simulink model "processor_with_peripherals"  (R2025a)
settings: Solver=FixedStepDiscrete  StartTime=0.0  StopTime=inf  RelTol=1e-3
libraries: simulink x6
(part 3 of 5)

== system processor_with_peripherals/SysTick_Timer ==
  In1 : Inport
  In2 : Inport  Port=2
  RAM_WData : Inport  Port=3
  Compare To Constant : simulink/Logic and Bit Operations/Compare To Constant  relop===  const=-16  OutDataTypeStr=boolean
  Counter Free-Running : simulink/Sources/Counter Free-Running  NumBits=16  tsamp=1
  Logical Operator : Logic  AllPortsSameDT=off  OutDataTypeStr=boolean
  Relational Operator : RelationalOperator  Operator===  OutDataTypeStr=boolean  RndMeth=Simplest  InputSameDT=off
  Scope : Scope
      settings: ActiveDisplayYMinimum=-1  ActiveDisplayYMaximum=1  DataLoggingVariableName=ScopeData7
  Switch : Switch  Criteria=u2 > Threshold  SaturateOnIntegerOverflow=off  InputSameDT=off
  Unit Delay : UnitDelay  InitialCondition=10000  HasFrameUpgradeWarning=on
  Out1 : Outport
  wires:
  In1/1 -> Compare To Constant/1  "Address"
  In2/1 -> Logical Operator/2  "MemWrite"
  RAM_WData/1 -> Switch/1  "WriteData"
  Relational Operator/1 -> Scope/1, Out1/1  "IRQ_Out"
  Compare To Constant/1 -> Logical Operator/1
  Unit Delay/1 -> Relational Operator/1, Switch/3
  Switch/1 -> Unit Delay/1
  Counter Free-Running/1 -> Relational Operator/2
  Logical Operator/1 -> Switch/2

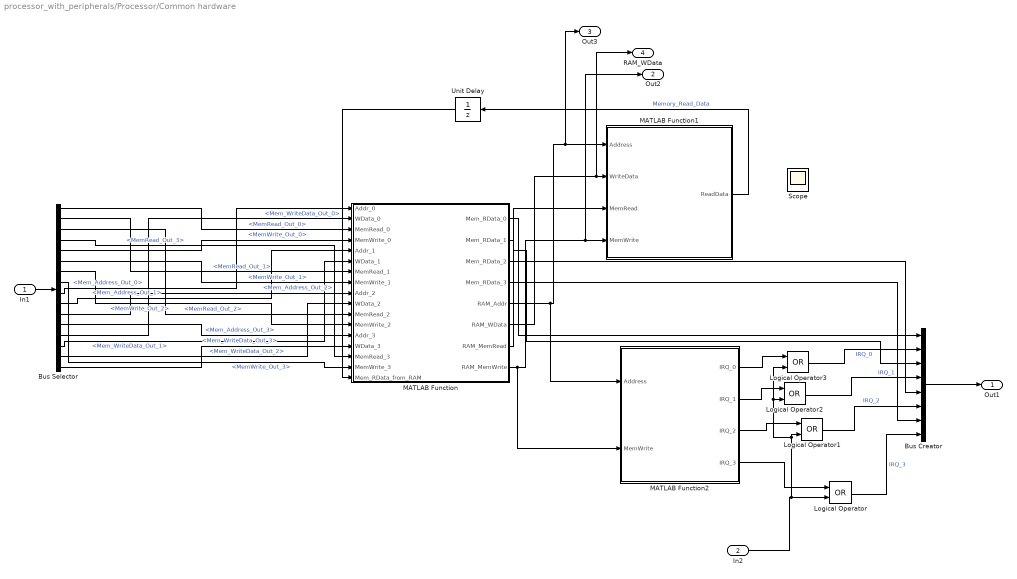
== system processor_with_peripherals/Processor/Common hardware ==
  In1 : Inport
  In2 : Inport  Port=2
  Bus Creator : BusCreator  Inputs=8  OutDataTypeStr=Bus: CH0_Bus
  Bus Selector : BusSelector  OutputSignals=MemRead_Out_0,MemRead_Out_1,MemRead_Out_2,MemRead_Out_3,MemWrite_Out_0,MemWrite_Out_1,MemWrite_Out_2,MemWrite_Out_3,Mem_Address_Out_0,Mem_Address_Out_1,Mem_Address_Out_2,Mem_Address_Out_3,Mem_WriteData_Out_0,Mem_WriteData_Out_1,Mem_WriteData_Out_2,Mem_WriteData_Out_3
  Logical Operator{,1..3} (4 alike) : Logic  Operator=OR  AllPortsSameDT=off  OutDataTypeStr=boolean
  MATLAB Function : MATLAB Function  TreatAsAtomicUnit=on
  MATLAB Function1 : MATLAB Function  TreatAsAtomicUnit=on
  MATLAB Function2 : MATLAB Function  TreatAsAtomicUnit=on
  Scope : Scope
      settings: ActiveDisplayYMinimum=-9.9596643418991722  ActiveDisplayYMaximum=10.040335658100835  DataLoggingVariableName=ScopeData3
  Unit Delay : UnitDelay  HasFrameUpgradeWarning=on
  Out1 : Outport
  Out2 : Outport  Port=2
  Out3 : Outport  Port=3
  RAM_WData : Outport  Port=4
  wires:
  MATLAB Function/5(RAM_Addr) -> MATLAB Function2/1(Address), Out3/1, MATLAB Function1/1(Address)
  MATLAB Function/6(RAM_WData) -> RAM_WData/1, MATLAB Function1/2(WriteData)
  MATLAB Function/7(RAM_MemRead) -> MATLAB Function1/3(MemRead)
  MATLAB Function/8(RAM_MemWrite) -> Out2/1, MATLAB Function1/4(MemWrite), MATLAB Function2/2(MemWrite)
  MATLAB Function1/1(ReadData) -> Unit Delay/1  "Memory_Read_Data"
  MATLAB Function/1(Mem_RData_0) -> Bus Creator/1
  MATLAB Function2/1(IRQ_0) -> Logical Operator3/1
  MATLAB Function/2(Mem_RData_1) -> Bus Creator/3
  MATLAB Function/3(Mem_RData_2) -> Bus Creator/5
  MATLAB Function2/3(IRQ_2) -> Logical Operator1/1
  MATLAB Function/4(Mem_RData_3) -> Bus Creator/7
  MATLAB Function2/4(IRQ_3) -> Logical Operator/1
  In1/1 -> Bus Selector/1
  Bus Creator/1 -> Out1/1
  Bus Selector/1 -> MATLAB Function/3(MemRead_0)  "<MemRead_Out_0>"
  Bus Selector/2 -> MATLAB Function/7(MemRead_1)  "<MemRead_Out_1>"
  Bus Selector/3 -> MATLAB Function/11(MemRead_2)  "<MemRead_Out_2>"
  Bus Selector/4 -> MATLAB Function/15(MemRead_3)  "<MemRead_Out_3>"
  Bus Selector/5 -> MATLAB Function/4(MemWrite_0)  "<MemWrite_Out_0>"
  Bus Selector/6 -> MATLAB Function/8(MemWrite_1)  "<MemWrite_Out_1>"
  Bus Selector/7 -> MATLAB Function/12(MemWrite_2)  "<MemWrite_Out_2>"
  Bus Selector/8 -> MATLAB Function/16(MemWrite_3)  "<MemWrite_Out_3>"
  Bus Selector/9 -> MATLAB Function/1(Addr_0)  "<Mem_Address_Out_0>"
  Bus Selector/10 -> MATLAB Function/5(Addr_1)  "<Mem_Address_Out_1>"
  Bus Selector/11 -> MATLAB Function/9(Addr_2)  "<Mem_Address_Out_2>"
  Bus Selector/12 -> MATLAB Function/13(Addr_3)  "<Mem_Address_Out_3>"
  Bus Selector/13 -> MATLAB Function/2(WData_0)  "<Mem_WriteData_Out_0>"
  Bus Selector/14 -> MATLAB Function/6(WData_1)  "<Mem_WriteData_Out_1>"
  Bus Selector/15 -> MATLAB Function/10(WData_2)  "<Mem_WriteData_Out_2>"
  Bus Selector/16 -> MATLAB Function/14(WData_3)  "<Mem_WriteData_Out_3>"
  Unit Delay/1 -> MATLAB Function/17(Mem_RData_from_RAM)
  Logical Operator/1 -> Bus Creator/8  "IRQ_3"
  Logical Operator1/1 -> Bus Creator/6  "IRQ_2"
  MATLAB Function2/2(IRQ_1) -> Logical Operator2/1
  Logical Operator2/1 -> Bus Creator/4  "IRQ_1"
  Logical Operator3/1 -> Bus Creator/2  "IRQ_0"
  In2/1 -> Logical Operator3/2, Logical Operator2/2, Logical Operator1/2, Logical Operator/2

== system processor_with_peripherals/Processor/Core_0 ==
  In1 : Inport
  In2 : Inport  Port=2
  Bus Creator : BusCreator  Inputs=10  OutDataTypeStr=Bus: C01_Bus
  Bus Selector : BusSelector  OutputSignals=Mem_RData_0,IRQ_0,Mem_RData_1,IRQ_1,Mem_RData_2,IRQ_2,Mem_RData_3,IRQ_3
  EX/MEM Pipeline Register : UnitDelay  HasFrameUpgradeWarning=on
  Execute (EX) Stage : Subsystem
  ID/EX Pipeline Register : UnitDelay  HasFrameUpgradeWarning=on
  IF/ID Pipeline Register : UnitDelay  HasFrameUpgradeWarning=on
  Instruction Decode(ID) Stage : Subsystem
  Instruction Fetch (IF) Stage : Subsystem
  MEM/WB Pipeline Register : UnitDelay  HasFrameUpgradeWarning=on
  Memory Access : Subsystem
  Write Back : Subsystem
  Out1 : Outport
  Out2 : Outport  Port=2
  wires:
  IF/ID Pipeline Register/1 -> Instruction Decode(ID) Stage/1(In1)
  Instruction Decode(ID) Stage/1(Out1) -> ID/EX Pipeline Register/1
  MEM/WB Pipeline Register/1 -> Write Back/1(In1)
  Memory Access/1(Out1) -> MEM/WB Pipeline Register/1
  Instruction Fetch (IF) Stage/1(Out1) -> IF/ID Pipeline Register/1
  EX/MEM Pipeline Register/1 -> Memory Access/1(In1)
  Execute (EX) Stage/1(Out1) -> EX/MEM Pipeline Register/1
  ID/EX Pipeline Register/1 -> Execute (EX) Stage/1(In1)
  Write Back/1(Out1) -> Instruction Decode(ID) Stage/2(In2)
  Instruction Fetch (IF) Stage/2(Out2) -> Out1/1  "Instruction_Address_Out"
  Memory Access/2(Out2) -> Bus Creator/3  "Mem_Address_Out_0"
  Memory Access/3(Out3) -> Bus Creator/2  "Mem_WriteData_Out_0"
  Memory Access/4(Out4) -> Bus Creator/1  "MemRead_Out_0"
  Memory Access/5(Out5) -> Bus Creator/4  "MemWrite_Out_0"
  Bus Selector/1 -> Write Back/2(In2)  "<Mem_RData_0>"
  In1/1 -> Bus Selector/1
  Bus Selector/2 -> Instruction Fetch (IF) Stage/2(In2)  "<IRQ_0>"
  Bus Creator/1 -> Out2/1
  Bus Selector/3 -> Bus Creator/5  "<Mem_RData_1>"
  Bus Selector/4 -> Bus Creator/6  "<IRQ_1>"
  Bus Selector/5 -> Bus Creator/7  "<Mem_RData_2>"
  Bus Selector/6 -> Bus Creator/8  "<IRQ_2>"
  Bus Selector/7 -> Bus Creator/9  "<Mem_RData_3>"
  Bus Selector/8 -> Bus Creator/10  "<IRQ_3>"
  In2/1 -> Instruction Fetch (IF) Stage/1(In1)

== system processor_with_peripherals/Processor/Core_1 ==
  In2 : Inport
  In1 : Inport  Port=2
  Bus Creator : BusCreator  Inputs=12  OutDataTypeStr=Bus: C12_Bus
  Bus Selector : BusSelector  OutputSignals=IRQ_1,Mem_RData_1,MemWrite_Out_0,Mem_Address_Out_0,Mem_WriteData_Out_0,MemRead_Out_0,Mem_RData_2,IRQ_2,Mem_RData_3,IRQ_3
  EX/MEM Pipeline Register : UnitDelay  HasFrameUpgradeWarning=on
  Execute (EX) Stage : Subsystem
  ID/EX Pipeline Register : UnitDelay  HasFrameUpgradeWarning=on
  IF/ID Pipeline Register : UnitDelay  HasFrameUpgradeWarning=on
  Instruction Decode(ID) Stage : Subsystem
  Instruction Fetch (IF) Stage : Subsystem
  MEM/WB Pipeline Register : UnitDelay  HasFrameUpgradeWarning=on
  Memory Access : Subsystem
  Write Back : Subsystem
  Out1 : Outport
  Out2 : Outport  Port=2
  wires:
  IF/ID Pipeline Register/1 -> Instruction Decode(ID) Stage/1(In1)
  Instruction Decode(ID) Stage/1(Out1) -> ID/EX Pipeline Register/1
  MEM/WB Pipeline Register/1 -> Write Back/1(In1)
  Memory Access/1(Out1) -> MEM/WB Pipeline Register/1
  Instruction Fetch (IF) Stage/1(Out1) -> IF/ID Pipeline Register/1
  EX/MEM Pipeline Register/1 -> Memory Access/1(In1)
  Execute (EX) Stage/1(Out1) -> EX/MEM Pipeline Register/1
  ID/EX Pipeline Register/1 -> Execute (EX) Stage/1(In1)
  Write Back/1(Out1) -> Instruction Decode(ID) Stage/2(In2)
  Instruction Fetch (IF) Stage/2(Out2) -> Out1/1  "Instruction_Address_Out"
  Memory Access/2(Out2) -> Bus Creator/3  "Mem_Address_Out_1"
  Memory Access/3(Out3) -> Bus Creator/2  "Mem_WriteData_Out_1"
  Memory Access/4(Out4) -> Bus Creator/1  "MemRead_Out_1"
  Memory Access/5(Out5) -> Bus Creator/4  "MemWrite_Out_1"
  In2/1 -> Bus Selector/1
  Bus Creator/1 -> Out2/1
  In1/1 -> Instruction Fetch (IF) Stage/1(In1)
  Bus Selector/1 -> Instruction Fetch (IF) Stage/2(In2)  "<IRQ_1>"
  Bus Selector/2 -> Write Back/2(In2)  "<Mem_RData_1>"
  Bus Selector/3 -> Bus Creator/5  "<MemWrite_Out_0>"
  Bus Selector/4 -> Bus Creator/6  "<Mem_Address_Out_0>"
  Bus Selector/5 -> Bus Creator/7  "<Mem_WriteData_Out_0>"
  Bus Selector/6 -> Bus Creator/8  "<MemRead_Out_0>"
  Bus Selector/7 -> Bus Creator/9  "<Mem_RData_2>"
  Bus Selector/8 -> Bus Creator/10  "<IRQ_2>"
  Bus Selector/9 -> Bus Creator/11  "<Mem_RData_3>"
  Bus Selector/10 -> Bus Creator/12  "<IRQ_3>"

== system processor_with_peripherals/Processor/Core_2 ==
  In1 : Inport
  In2 : Inport  Port=2
  Bus Creator : BusCreator  Inputs=14  OutDataTypeStr=Bus: C23_Bus
  Bus Selector : BusSelector  OutputSignals=Mem_RData_2,IRQ_2,MemRead_Out_1,Mem_WriteData_Out_1,Mem_Address_Out_1,MemWrite_Out_1,MemWrite_Out_0,Mem_Address_Out_0,Mem_WriteData_Out_0,MemRead_Out_0,Mem_RData_3,IRQ_3
  EX/MEM Pipeline Register : UnitDelay  HasFrameUpgradeWarning=on
  Execute (EX) Stage : Subsystem
  ID/EX Pipeline Register : UnitDelay  HasFrameUpgradeWarning=on
  IF/ID Pipeline Register : UnitDelay  HasFrameUpgradeWarning=on
  Instruction Decode(ID) Stage : Subsystem
  Instruction Fetch (IF) Stage : Subsystem
  MEM/WB Pipeline Register : UnitDelay  HasFrameUpgradeWarning=on
  Memory Access : Subsystem
  Write Back : Subsystem
  Out1 : Outport
  Out2 : Outport  Port=2
  wires:
  IF/ID Pipeline Register/1 -> Instruction Decode(ID) Stage/1(In1)
  Instruction Decode(ID) Stage/1(Out1) -> ID/EX Pipeline Register/1
  MEM/WB Pipeline Register/1 -> Write Back/1(In1)
  Memory Access/1(Out1) -> MEM/WB Pipeline Register/1
  Instruction Fetch (IF) Stage/1(Out1) -> IF/ID Pipeline Register/1
  EX/MEM Pipeline Register/1 -> Memory Access/1(In1)
  Execute (EX) Stage/1(Out1) -> EX/MEM Pipeline Register/1
  ID/EX Pipeline Register/1 -> Execute (EX) Stage/1(In1)
  Write Back/1(Out1) -> Instruction Decode(ID) Stage/2(In2)
  In1/1 -> Instruction Fetch (IF) Stage/1(In1)  "Instruction_In"
  Instruction Fetch (IF) Stage/2(Out2) -> Out1/1  "Instruction_Address_Out"
  Memory Access/2(Out2) -> Bus Creator/3  "Mem_Address_Out_2"
  Memory Access/3(Out3) -> Bus Creator/2  "Mem_WriteData_Out_2"
  Memory Access/4(Out4) -> Bus Creator/1  "MemRead_Out_2"
  Memory Access/5(Out5) -> Bus Creator/4  "MemWrite_Out_2"
  Bus Selector/1 -> Write Back/2(In2)  "<Mem_RData_2>"
  Bus Selector/2 -> Instruction Fetch (IF) Stage/2(In2)  "<IRQ_2>"
  In2/1 -> Bus Selector/1
  Bus Creator/1 -> Out2/1
  Bus Selector/3 -> Bus Creator/5  "<MemRead_Out_1>"
  Bus Selector/4 -> Bus Creator/6  "<Mem_WriteData_Out_1>"
  Bus Selector/5 -> Bus Creator/7  "<Mem_Address_Out_1>"
  Bus Selector/6 -> Bus Creator/8  "<MemWrite_Out_1>"
  Bus Selector/7 -> Bus Creator/9  "<MemWrite_Out_0>"
  Bus Selector/8 -> Bus Creator/10  "<Mem_Address_Out_0>"
  Bus Selector/9 -> Bus Creator/11  "<Mem_WriteData_Out_0>"
  Bus Selector/10 -> Bus Creator/12  "<MemRead_Out_0>"
  Bus Selector/11 -> Bus Creator/13  "<Mem_RData_3>"
  Bus Selector/12 -> Bus Creator/14  "<IRQ_3>"

== system processor_with_peripherals/Processor/Core_3 ==
  In1 : Inport
  In2 : Inport  Port=2
  Bus Creator : BusCreator  Inputs=16  OutDataTypeStr=Bus: C3CH_Bus
  Bus Selector : BusSelector  OutputSignals=IRQ_3,Mem_RData_3,MemRead_Out_1,MemWrite_Out_2,Mem_Address_Out_2,Mem_WriteData_Out_2,MemRead_Out_2,Mem_WriteData_Out_1,Mem_Address_Out_1,MemWrite_Out_1,MemWrite_Out_0,Mem_Address_Out_0,Mem_WriteData_Out_0,MemRead_Out_0
  EX/MEM Pipeline Register : UnitDelay  HasFrameUpgradeWarning=on
  Execute (EX) Stage : Subsystem
  ID/EX Pipeline Register : UnitDelay  HasFrameUpgradeWarning=on
  IF/ID Pipeline Register : UnitDelay  HasFrameUpgradeWarning=on
  Instruction Decode(ID) Stage : Subsystem
  Instruction Fetch (IF) Stage : Subsystem
  MEM/WB Pipeline Register : UnitDelay  HasFrameUpgradeWarning=on
  Memory Access : Subsystem
  Write Back : Subsystem
  Out1 : Outport
  Out2 : Outport  Port=2
  wires:
  IF/ID Pipeline Register/1 -> Instruction Decode(ID) Stage/1(In1)
  Instruction Decode(ID) Stage/1(Out1) -> ID/EX Pipeline Register/1
  MEM/WB Pipeline Register/1 -> Write Back/1(In1)
  Memory Access/1(Out1) -> MEM/WB Pipeline Register/1
  Instruction Fetch (IF) Stage/1(Out1) -> IF/ID Pipeline Register/1
  EX/MEM Pipeline Register/1 -> Memory Access/1(In1)
  Execute (EX) Stage/1(Out1) -> EX/MEM Pipeline Register/1
  ID/EX Pipeline Register/1 -> Execute (EX) Stage/1(In1)
  Write Back/1(Out1) -> Instruction Decode(ID) Stage/2(In2)
  In1/1 -> Instruction Fetch (IF) Stage/1(In1)  "Instruction_In"
  Instruction Fetch (IF) Stage/2(Out2) -> Out1/1  "Instruction_Address_Out"
  Memory Access/2(Out2) -> Bus Creator/3  "Mem_Address_Out_3"
  Memory Access/3(Out3) -> Bus Creator/2  "Mem_WriteData_Out_3"
  Memory Access/4(Out4) -> Bus Creator/1  "MemRead_Out_3"
  Memory Access/5(Out5) -> Bus Creator/4  "MemWrite_Out_3"
  Bus Selector/2 -> Write Back/2(In2)  "<Mem_RData_3>"
  In2/1 -> Bus Selector/1
  Bus Creator/1 -> Out2/1
  Bus Selector/1 -> Instruction Fetch (IF) Stage/2(In2)  "<IRQ_3>"
  Bus Selector/3 -> Bus Creator/5  "<MemRead_Out_1>"
  Bus Selector/4 -> Bus Creator/6  "<MemWrite_Out_2>"
  Bus Selector/5 -> Bus Creator/7  "<Mem_Address_Out_2>"
  Bus Selector/6 -> Bus Creator/8  "<Mem_WriteData_Out_2>"
  Bus Selector/7 -> Bus Creator/9  "<MemRead_Out_2>"
  Bus Selector/8 -> Bus Creator/10  "<Mem_WriteData_Out_1>"
  Bus Selector/9 -> Bus Creator/11  "<Mem_Address_Out_1>"
  Bus Selector/10 -> Bus Creator/12  "<MemWrite_Out_1>"
  Bus Selector/11 -> Bus Creator/13  "<MemWrite_Out_0>"
  Bus Selector/12 -> Bus Creator/14  "<Mem_Address_Out_0>"
  Bus Selector/13 -> Bus Creator/15  "<Mem_WriteData_Out_0>"
  Bus Selector/14 -> Bus Creator/16  "<MemRead_Out_0>"

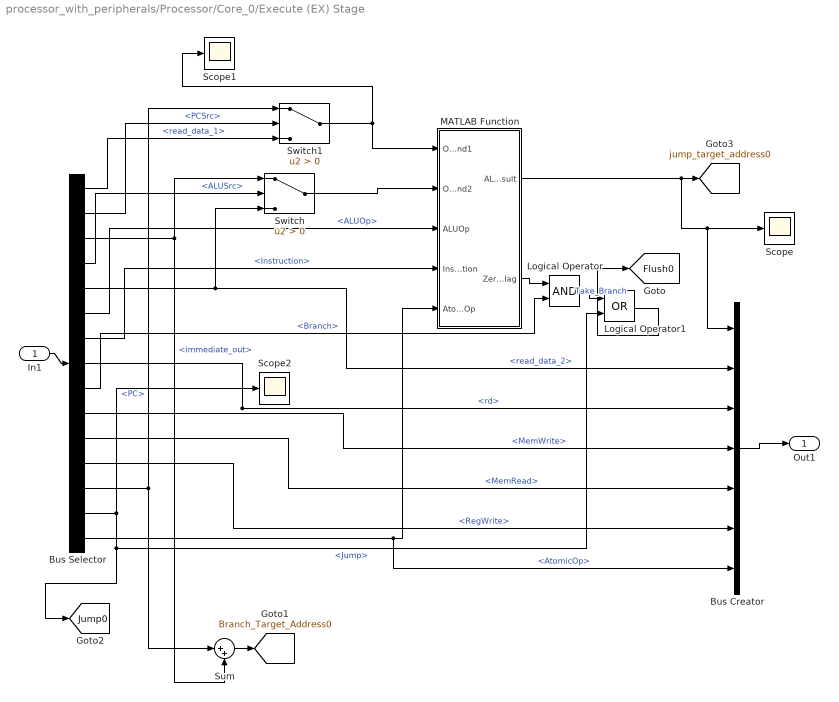
== system processor_with_peripherals/Processor/Core_0/Execute (EX) Stage ==
  In1 : Inport
  Bus Creator : BusCreator  Inputs=7  OutDataTypeStr=Bus: EXMEM_Bus  NonVirtualBus=on
  Bus Selector : BusSelector  OutputSignals=read_data_1,PCSrc,immediate_out,ALUSrc,read_data_2,ALUOp,Instruction,rd,Branch,MemWrite,MemRead,RegWrite,PC,Jump,AtomicOp
  Logical Operator : Logic  AllPortsSameDT=off  OutDataTypeStr=boolean
  Logical Operator1 : Logic  Operator=OR  AllPortsSameDT=off  OutDataTypeStr=boolean
  MATLAB Function : MATLAB Function  TreatAsAtomicUnit=on
  Scope : Scope
      settings: ActiveDisplayYMinimum=31.795159975888414  ActiveDisplayYMaximum=57.507794048249679
  Scope1 : Scope
      settings: ActiveDisplayYMinimum=91.787947621079041  ActiveDisplayYMaximum=102.5794088339111
  Scope2 : Scope
      settings: ActiveDisplayYMinimum=-11.618054609297872  ActiveDisplayYMaximum=8.6667189404735723  DataLoggingVariableName=ScopeData2
  Sum : Sum  Inputs=|++
  Switch : Switch  Criteria=u2 > Threshold  OutDataTypeStr=int32  SaturateOnIntegerOverflow=off  InputSameDT=off
  Switch1 : Switch  Criteria=u2 > Threshold  OutDataTypeStr=int32  SaturateOnIntegerOverflow=off  InputSameDT=off
  Out1 : Outport
  tag scope: Branch_Target_Address0=global, Flush0=global, Jump0=global, jump_target_address0=global
  wires:
  Bus Creator/1 -> Out1/1
  In1/1 -> Bus Selector/1
  Bus Selector/3 -> Sum/2, Switch/1  "<immediate_out>"
  Bus Selector/8 -> Bus Creator/3  "<rd>"
  Bus Selector/5 -> Bus Creator/2, Switch/3  "<read_data_2>"
  Bus Selector/1 -> Switch1/3  "<read_data_1>"
  Bus Selector/6 -> MATLAB Function/3(ALUOp)  "<ALUOp>"
  Bus Selector/14 -> [Jump0], Logical Operator1/2, Scope2/1  "<Jump>"
  Bus Selector/9 -> Logical Operator/2  "<Branch>"
  Bus Selector/10 -> Bus Creator/4  "<MemWrite>"
  Bus Selector/11 -> Bus Creator/5  "<MemRead>"
  Bus Selector/4 -> Switch/2  "<ALUSrc>"
  Bus Selector/12 -> Bus Creator/6  "<RegWrite>"
  Bus Selector/7 -> MATLAB Function/4(Instruction)  "<Instruction>"
  Switch/1 -> MATLAB Function/2(Operand2)
  MATLAB Function/1(ALU_Result) -> Scope/1, Bus Creator/1, [jump_target_address0]
  MATLAB Function/2(Zero_Flag) -> Logical Operator/1
  Logical Operator/1 -> Logical Operator1/1  "Take_Branch"
  Bus Selector/13 -> Sum/1, Switch1/1  "<PC>"
  Sum/1 -> [Branch_Target_Address0]
  Bus Selector/2 -> Switch1/2  "<PCSrc>"
  Switch1/1 -> Scope1/1, MATLAB Function/1(Operand1)
  Logical Operator1/1 -> [Flush0]
  Bus Selector/15 -> Bus Creator/7, MATLAB Function/5(AtomicOp)  "<AtomicOp>"

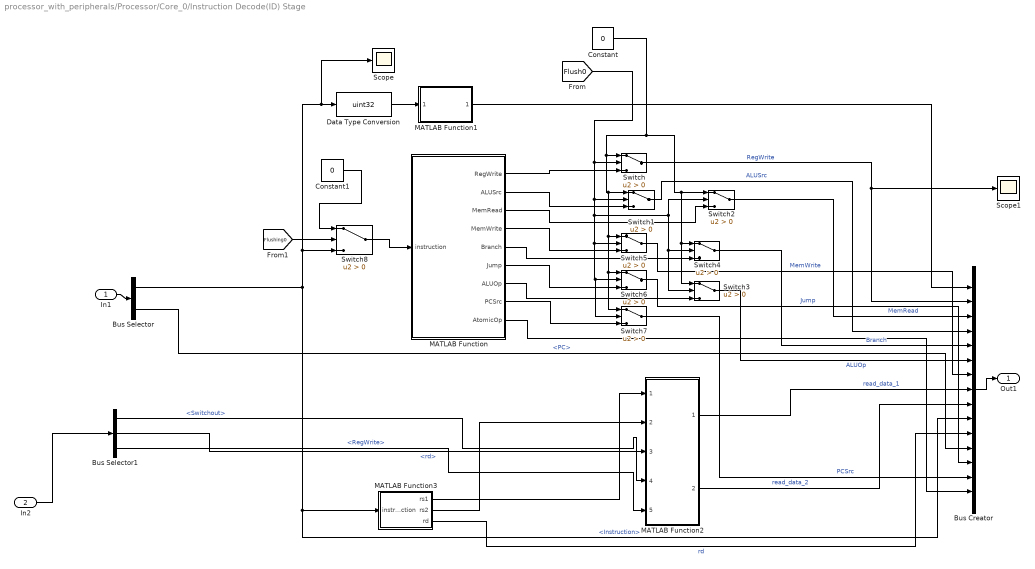
== system processor_with_peripherals/Processor/Core_0/Instruction Decode(ID) Stage ==
  In1 : Inport
  In2 : Inport  Port=2
  Bus Creator : BusCreator  Inputs=15  OutDataTypeStr=Bus: IDEX_Bus  NonVirtualBus=on
  Bus Selector : BusSelector  OutputSignals=Instruction,PC
  Bus Selector1 : BusSelector  OutputSignals=Switchout,rd,RegWrite
  Constant : Constant  Value=0  OutDataTypeStr=uint8
  Constant1 : Constant  Value=0
  Data Type Conversion : DataTypeConversion  OutDataTypeStr=uint32  SaturateOnIntegerOverflow=off  RndMeth=Floor
  MATLAB Function : MATLAB Function  TreatAsAtomicUnit=on
  MATLAB Function1 : MATLAB Function  TreatAsAtomicUnit=on
  MATLAB Function2 : MATLAB Function  TreatAsAtomicUnit=on
  MATLAB Function3 : MATLAB Function  TreatAsAtomicUnit=on
  Scope : Scope
      settings: ActiveDisplayYMinimum=-8.6059552101299882E+7  ActiveDisplayYMaximum=2.8669047582629967E+8  DataLoggingVariableName=ScopeData4
  Scope1 : Scope
      settings: ActiveDisplayYMinimum=-20.131283374012085  ActiveDisplayYMaximum=16.717122271781463  DataLoggingVariableName=ScopeData5
  Switch{,1..2,5..6} (5 alike) : Switch  Criteria=u2 > Threshold  OutDataTypeStr=boolean  SaturateOnIntegerOverflow=off  InputSameDT=off
  Switch3 : Switch  Criteria=u2 > Threshold  OutDataTypeStr=uint32  SaturateOnIntegerOverflow=off  InputSameDT=off
  Switch4 : Switch  Criteria=u2 > Threshold  OutDataTypeStr=uint32  SaturateOnIntegerOverflow=off  InputSameDT=off
  Switch7 : Switch  Criteria=u2 > Threshold  OutDataTypeStr=uint32  SaturateOnIntegerOverflow=off  InputSameDT=off
  Switch8 : Switch  Criteria=u2 > Threshold  SaturateOnIntegerOverflow=off  InputSameDT=off
  Out1 : Outport
  wires:
  Bus Creator/1 -> Out1/1
  In1/1 -> Bus Selector/1
  Bus Selector/1 -> Data Type Conversion/1, Scope/1, Switch8/3, MATLAB Function3/1(instruction), Bus Creator/10  "<Instruction>"
  MATLAB Function2/1(ReadData1) -> Bus Creator/8  "read_data_1"
  MATLAB Function2/2(ReadData2) -> Bus Creator/9  "read_data_2"
  MATLAB Function1/1(immediate_out) -> Bus Creator/1
  MATLAB Function3/3(rd) -> Bus Creator/11  "rd"
  MATLAB Function/7(ALUOp) -> Switch3/3
  MATLAB Function/6(Jump) -> Switch6/3
  MATLAB Function/5(Branch) -> Switch4/3
  MATLAB Function/4(MemWrite) -> Switch5/3
  MATLAB Function/3(MemRead) -> Switch2/3
  MATLAB Function/2(ALUSrc) -> Switch1/3
  Bus Selector1/2 -> MATLAB Function2/3(WriteAddr)  "<rd>"
  Bus Selector1/3 -> MATLAB Function2/5(WriteEnable)  "<RegWrite>"
  Bus Selector1/1 -> MATLAB Function2/4(WriteData)  "<Switchout>"
  MATLAB Function3/2(rs2) -> MATLAB Function2/2(ReadAddr2)
  Bus Selector/2 -> Bus Creator/12  "<PC>"
  MATLAB Function/8(PCSrc) -> Switch7/3
  MATLAB Function/1(RegWrite) -> Switch/3
  [Flush0] -> Switch1/2, Switch3/2, Switch4/2, Switch2/2, Switch7/2, Switch6/2, Switch5/2, Switch/2
  Constant/1 -> Switch3/1, Switch4/1, Switch2/1, Switch7/1, Switch6/1, Switch5/1, Switch1/1, Switch/1
  Switch/1 -> Scope1/1, Bus Creator/2  "RegWrite"
  Switch2/1 -> Bus Creator/3  "MemRead"
  Switch1/1 -> Bus Creator/4  "ALUSrc"
  Switch4/1 -> Bus Creator/5  "Branch"
  Switch3/1 -> Bus Creator/6  "ALUOp"
  Switch5/1 -> Bus Creator/7  "MemWrite"
  Switch6/1 -> Bus Creator/13  "Jump"
  Switch7/1 -> Bus Creator/14  "PCSrc"
  MATLAB Function3/1(rs1) -> MATLAB Function2/1(ReadAddr1)
  In2/1 -> Bus Selector1/1
  Switch8/1 -> MATLAB Function/1(instruction)
  Constant1/1 -> Switch8/1
  [Flushing0] -> Switch8/2
  Data Type Conversion/1 -> MATLAB Function1/1(instruction)
  MATLAB Function/9(AtomicOp) -> Bus Creator/15

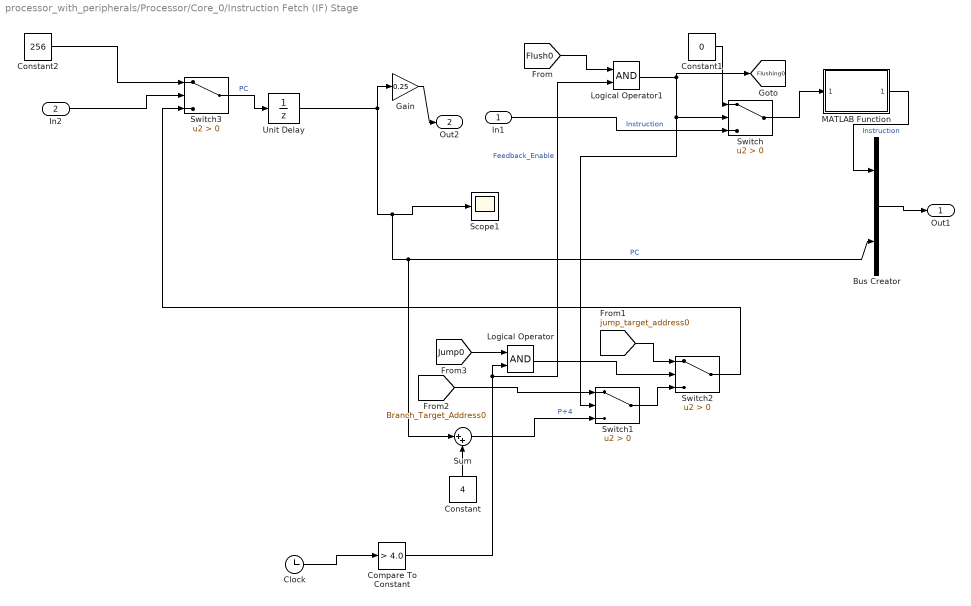
== system processor_with_peripherals/Processor/Core_0/Instruction Fetch (IF) Stage ==
  In1 : Inport
  In2 : Inport  Port=2
  Bus Creator : BusCreator  Inputs=2  OutDataTypeStr=Bus: IFID_Bus  NonVirtualBus=on
  Clock : Clock
  Compare To Constant : simulink/Logic and Bit Operations/Compare To Constant  relop=>  const=4.0  OutDataTypeStr=boolean
  Constant : Constant  Value=4
  Constant1 : Constant  Value=0
  Constant2 : Constant  Value=256  OutDataTypeStr=uint32
  Gain : Gain  Gain=0.25  OutDataTypeStr=uint32
  Logical Operator : Logic  AllPortsSameDT=off  OutDataTypeStr=boolean
  Logical Operator1 : Logic  AllPortsSameDT=off  OutDataTypeStr=boolean
  MATLAB Function : MATLAB Function  TreatAsAtomicUnit=on
  Scope1 : Scope
      settings: ActiveDisplayYMinimum=14.083038013644533  ActiveDisplayYMaximum=56.284353840527714  DataLoggingVariableName=ScopeData6
  Sum : Sum  Inputs=|++  OutDataTypeStr=uint32  AccumDataTypeStr=uint32
  Switch : Switch  Criteria=u2 > Threshold  OutDataTypeStr=uint32  SaturateOnIntegerOverflow=off  InputSameDT=off
  Switch1 : Switch  Criteria=u2 > Threshold  OutDataTypeStr=uint32  SaturateOnIntegerOverflow=off  InputSameDT=off
  Switch2 : Switch  Criteria=u2 > Threshold  OutDataTypeStr=uint32  SaturateOnIntegerOverflow=off  InputSameDT=off
  Switch3 : Switch  Criteria=u2 > Threshold  SaturateOnIntegerOverflow=off  InputSameDT=off
  Unit Delay : UnitDelay  HasFrameUpgradeWarning=on
  Out1 : Outport
  Out2 : Outport  Port=2
  tag scope: Flushing0=global
  wires:
  Switch3/1 -> Unit Delay/1  "PC"
  Constant/1 -> Sum/2
  In1/1 -> Switch/3  "Instruction"
  [jump_target_address0] -> Switch2/1
  Logical Operator1/1 -> Switch/2, Switch1/2, [Flushing0]
  Sum/1 -> Switch1/3  "P+4"
  Bus Creator/1 -> Out1/1
  Switch1/1 -> Switch2/3
  Switch2/1 -> Switch3/3
  [Jump0] -> Logical Operator/1
  [Branch_Target_Address0] -> Switch1/1
  Clock/1 -> Compare To Constant/1
  Compare To Constant/1 -> Logical Operator1/2, Logical Operator/2  "Feedback_Enable"
  Logical Operator/1 -> Switch2/2
  [Flush0] -> Logical Operator1/1
  MATLAB Function/1(scalar_out) -> Bus Creator/1  "Instruction"
  Switch/1 -> MATLAB Function/1(vector_in)
  Constant1/1 -> Switch/1
  Gain/1 -> Out2/1
  Constant2/1 -> Switch3/1
  In2/1 -> Switch3/2
  Unit Delay/1 -> Scope1/1, Bus Creator/2, Sum/1, Gain/1  "PC"

== system processor_with_peripherals/Processor/Core_0/Memory Access ==
  In1 : Inport
  Bus Creator : BusCreator  Inputs=4  OutDataTypeStr=Bus: MEMWB_Bus
  Bus Selector : BusSelector  OutputSignals=read_data_2,ALU_Result,MemWrite,RegWrite,MemRead,rd,AtomicOp
  Switch : Switch  Criteria=u2 > Threshold  SaturateOnIntegerOverflow=off  InputSameDT=off
  Out1 : Outport
  Out2 : Outport  Port=2
  Out3 : Outport  Port=3
  Out4 : Outport  Port=4
  Out5 : Outport  Port=5
  wires:
  In1/1 -> Bus Selector/1
  Bus Selector/2 -> Switch/1, Out2/1, Bus Creator/1  "<ALU_Result>"
  Bus Selector/6 -> Bus Creator/4  "<rd>"
  Bus Selector/3 -> Out5/1  "<MemWrite>"
  Bus Selector/5 -> Bus Creator/3, Out4/1  "<MemRead>"
  Bus Selector/4 -> Bus Creator/2  "<RegWrite>"
  Bus Selector/1 -> Switch/3  "<read_data_2>"
  Bus Creator/1 -> Out1/1
  Switch/1 -> Out3/1
  Bus Selector/7 -> Switch/2  "<AtomicOp>"

== system processor_with_peripherals/Processor/Core_0/Write Back ==
  In1 : Inport
  In2 : Inport  Port=2
  Bus Creator : BusCreator  Inputs=3
  Bus Selector : BusSelector  OutputSignals=ALU_Result,rd,MemRead,RegWrite
  Switch : Switch  Criteria=u2 > Threshold  SaturateOnIntegerOverflow=off  InputSameDT=off
  Out1 : Outport
  wires:
  Bus Creator/1 -> Out1/1
  In1/1 -> Bus Selector/1
  Bus Selector/1 -> Switch/3  "<ALU_Result>"
  Bus Selector/2 -> Bus Creator/2  "<rd>"
  Bus Selector/4 -> Bus Creator/3  "<RegWrite>"
  Bus Selector/3 -> Switch/2  "<MemRead>"
  Switch/1 -> Bus Creator/1  "Switchout"
  In2/1 -> Switch/1

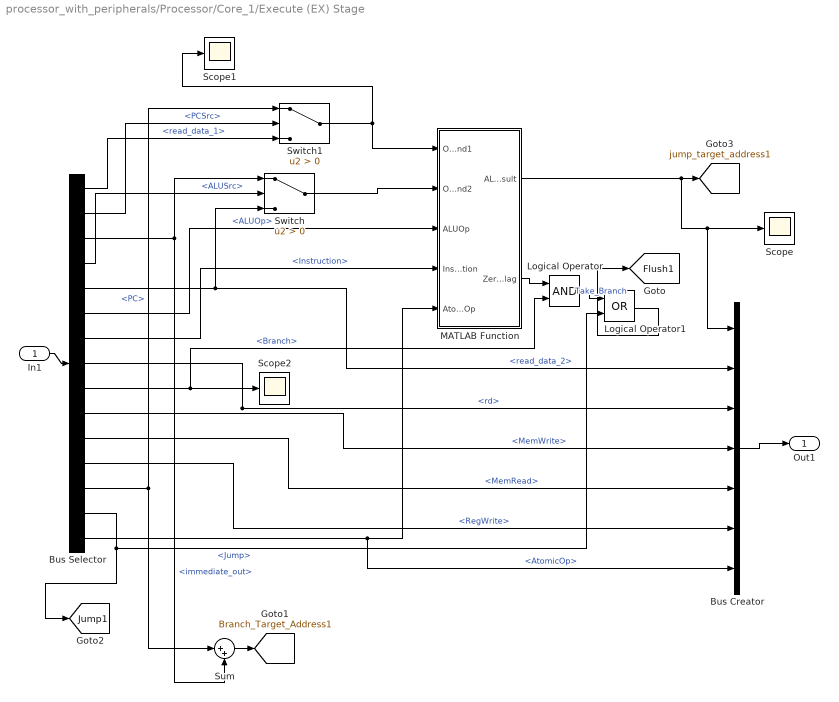
== system processor_with_peripherals/Processor/Core_1/Execute (EX) Stage ==
  In1 : Inport
  Bus Creator : BusCreator  Inputs=7  OutDataTypeStr=Bus: EXMEM_Bus  NonVirtualBus=on
  Bus Selector : BusSelector  OutputSignals=read_data_1,PCSrc,immediate_out,ALUSrc,read_data_2,ALUOp,Instruction,rd,Branch,MemWrite,MemRead,RegWrite,PC,Jump,AtomicOp
  Logical Operator : Logic  AllPortsSameDT=off  OutDataTypeStr=boolean
  Logical Operator1 : Logic  Operator=OR  AllPortsSameDT=off  OutDataTypeStr=boolean
  MATLAB Function : MATLAB Function  TreatAsAtomicUnit=on
  Scope : Scope
      settings: ActiveDisplayYMinimum=-21071.2731849412  ActiveDisplayYMaximum=99909.748218819586
  Scope1 : Scope
      settings: ActiveDisplayYMinimum=91.787947621079041  ActiveDisplayYMaximum=102.5794088339111
  Scope2 : Scope
      settings: ActiveDisplayYMinimum=-10.291310820308553  ActiveDisplayYMaximum=8.1075767531802825  DataLoggingVariableName=ScopeData2
  Sum : Sum  Inputs=|++
  Switch : Switch  Criteria=u2 > Threshold  OutDataTypeStr=int32  SaturateOnIntegerOverflow=off  InputSameDT=off
  Switch1 : Switch  Criteria=u2 > Threshold  OutDataTypeStr=int32  SaturateOnIntegerOverflow=off  InputSameDT=off
  Out1 : Outport
  tag scope: Branch_Target_Address1=global, Flush1=global, Jump1=global, jump_target_address1=global
  wires:
  Bus Creator/1 -> Out1/1
  In1/1 -> Bus Selector/1
  Bus Selector/3 -> Sum/2, Switch/1  "<immediate_out>"
  Bus Selector/8 -> Bus Creator/3  "<rd>"
  Bus Selector/5 -> Bus Creator/2, Switch/3  "<read_data_2>"
  Bus Selector/1 -> Switch1/3  "<read_data_1>"
  Bus Selector/6 -> MATLAB Function/3(ALUOp)  "<ALUOp>"
  Bus Selector/14 -> [Jump1], Logical Operator1/2  "<Jump>"
  Bus Selector/9 -> Logical Operator/2, Scope2/1  "<Branch>"
  Bus Selector/10 -> Bus Creator/4  "<MemWrite>"
  Bus Selector/11 -> Bus Creator/5  "<MemRead>"
  Bus Selector/4 -> Switch/2  "<ALUSrc>"
  Bus Selector/12 -> Bus Creator/6  "<RegWrite>"
  Bus Selector/7 -> MATLAB Function/4(Instruction)  "<Instruction>"
  Switch/1 -> MATLAB Function/2(Operand2)
  MATLAB Function/1(ALU_Result) -> Scope/1, Bus Creator/1, [jump_target_address1]
  MATLAB Function/2(Zero_Flag) -> Logical Operator/1
  Logical Operator/1 -> Logical Operator1/1  "Take_Branch"
  Bus Selector/13 -> Sum/1, Switch1/1  "<PC>"
  Sum/1 -> [Branch_Target_Address1]
  Bus Selector/2 -> Switch1/2  "<PCSrc>"
  Switch1/1 -> Scope1/1, MATLAB Function/1(Operand1)
  Logical Operator1/1 -> [Flush1]
  Bus Selector/15 -> Bus Creator/7, MATLAB Function/5(AtomicOp)  "<AtomicOp>"

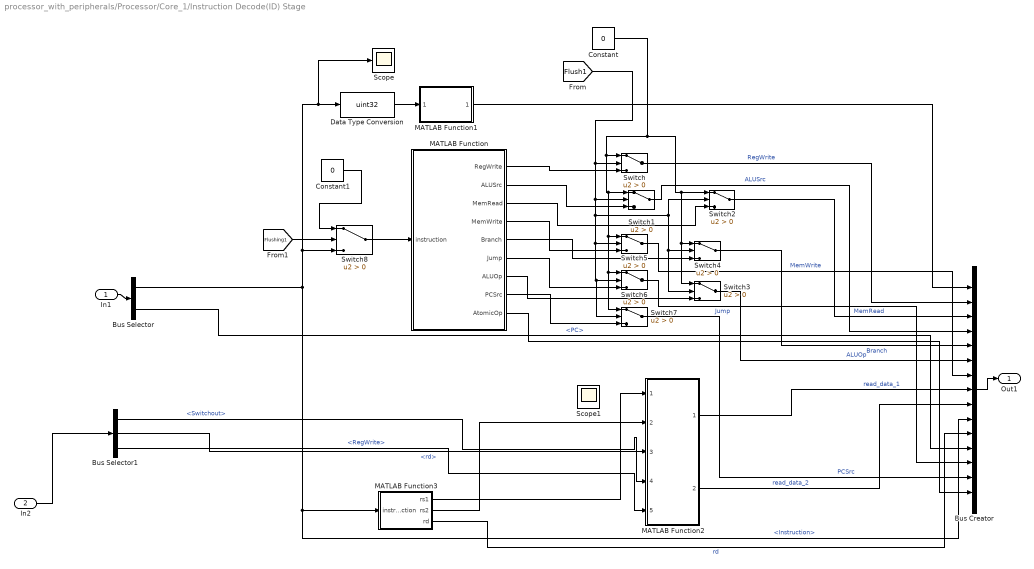
== system processor_with_peripherals/Processor/Core_1/Instruction Decode(ID) Stage ==
  In1 : Inport
  In2 : Inport  Port=2
  Bus Creator : BusCreator  Inputs=15  OutDataTypeStr=Bus: IDEX_Bus  NonVirtualBus=on
  Bus Selector : BusSelector  OutputSignals=Instruction,PC
  Bus Selector1 : BusSelector  OutputSignals=Switchout,rd,RegWrite
  Constant : Constant  Value=0  OutDataTypeStr=uint8
  Constant1 : Constant  Value=0
  Data Type Conversion : DataTypeConversion  OutDataTypeStr=uint32  SaturateOnIntegerOverflow=off  RndMeth=Floor
  MATLAB Function : MATLAB Function  TreatAsAtomicUnit=on
  MATLAB Function1 : MATLAB Function  TreatAsAtomicUnit=on
  MATLAB Function2 : MATLAB Function  TreatAsAtomicUnit=on
  MATLAB Function3 : MATLAB Function  TreatAsAtomicUnit=on
  Scope : Scope
      settings: ActiveDisplayYMinimum=-8.6059552101299882E+7  ActiveDisplayYMaximum=2.8669047582629967E+8  DataLoggingVariableName=ScopeData4
  Scope1 : Scope
      settings: ActiveDisplayYMinimum=-1.0224235765954815E+6  ActiveDisplayYMaximum=2.6269684460485624E+6  DataLoggingVariableName=ScopeData5
  Switch{,1..2,5..6} (5 alike) : Switch  Criteria=u2 > Threshold  OutDataTypeStr=boolean  SaturateOnIntegerOverflow=off  InputSameDT=off
  Switch3 : Switch  Criteria=u2 > Threshold  OutDataTypeStr=uint32  SaturateOnIntegerOverflow=off  InputSameDT=off
  Switch4 : Switch  Criteria=u2 > Threshold  OutDataTypeStr=uint32  SaturateOnIntegerOverflow=off  InputSameDT=off
  Switch7 : Switch  Criteria=u2 > Threshold  OutDataTypeStr=uint32  SaturateOnIntegerOverflow=off  InputSameDT=off
  Switch8 : Switch  Criteria=u2 > Threshold  SaturateOnIntegerOverflow=off  InputSameDT=off
  Out1 : Outport
  wires:
  Bus Creator/1 -> Out1/1
  In1/1 -> Bus Selector/1
  Bus Selector/1 -> Data Type Conversion/1, Scope/1, Switch8/3, MATLAB Function3/1(instruction), Bus Creator/10  "<Instruction>"
  MATLAB Function2/1(ReadData1) -> Bus Creator/8  "read_data_1"
  MATLAB Function2/2(ReadData2) -> Bus Creator/9  "read_data_2"
  MATLAB Function1/1(immediate_out) -> Bus Creator/1
  MATLAB Function3/3(rd) -> Bus Creator/11  "rd"
  MATLAB Function/7(ALUOp) -> Switch3/3
  MATLAB Function/6(Jump) -> Switch6/3
  MATLAB Function/5(Branch) -> Switch4/3
  MATLAB Function/4(MemWrite) -> Switch5/3
  MATLAB Function/3(MemRead) -> Switch2/3
  MATLAB Function/2(ALUSrc) -> Switch1/3
  Bus Selector1/2 -> MATLAB Function2/3(WriteAddr)  "<rd>"
  Bus Selector1/3 -> MATLAB Function2/5(WriteEnable)  "<RegWrite>"
  Bus Selector1/1 -> MATLAB Function2/4(WriteData)  "<Switchout>"
  MATLAB Function3/2(rs2) -> MATLAB Function2/2(ReadAddr2)
  Bus Selector/2 -> Bus Creator/12  "<PC>"
  MATLAB Function/8(PCSrc) -> Switch7/3
  MATLAB Function/1(RegWrite) -> Switch/3
  [Flush1] -> Switch1/2, Switch3/2, Switch4/2, Switch2/2, Switch7/2, Switch6/2, Switch5/2, Switch/2
  Constant/1 -> Switch3/1, Switch4/1, Switch2/1, Switch7/1, Switch6/1, Switch5/1, Switch1/1, Switch/1
  Switch/1 -> Bus Creator/2  "RegWrite"
  Switch2/1 -> Bus Creator/3  "MemRead"
  Switch1/1 -> Bus Creator/4  "ALUSrc"
  Switch4/1 -> Bus Creator/5  "Branch"
  Switch3/1 -> Bus Creator/6  "ALUOp"
  Switch5/1 -> Bus Creator/7  "MemWrite"
  Switch6/1 -> Bus Creator/13  "Jump"
  Switch7/1 -> Bus Creator/14  "PCSrc"
  MATLAB Function3/1(rs1) -> MATLAB Function2/1(ReadAddr1)
  In2/1 -> Bus Selector1/1
  Switch8/1 -> MATLAB Function/1(instruction)
  Constant1/1 -> Switch8/1
  [Flushing1] -> Switch8/2
  Data Type Conversion/1 -> MATLAB Function1/1(instruction)
  MATLAB Function/9(AtomicOp) -> Bus Creator/15

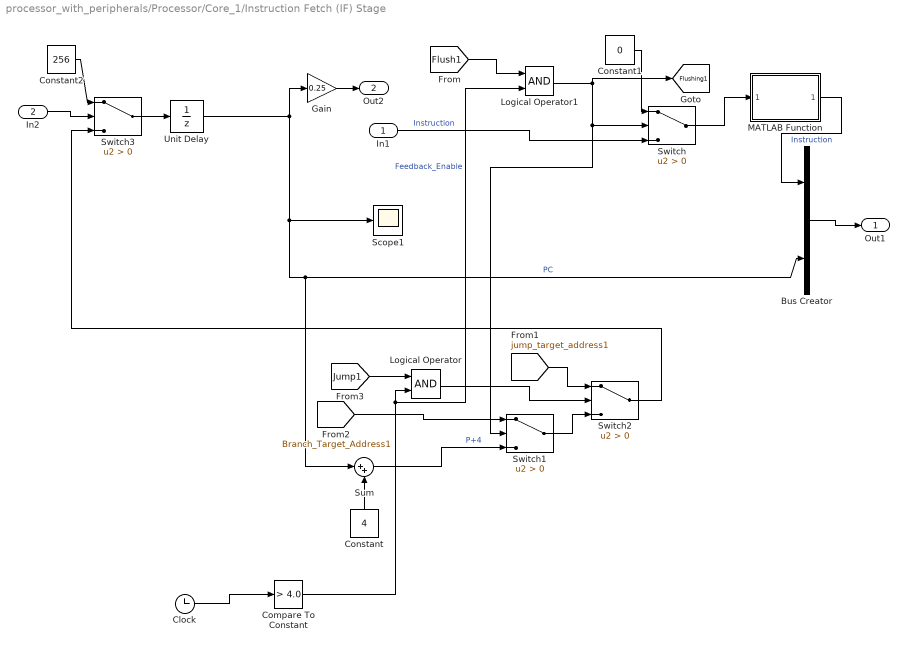
== system processor_with_peripherals/Processor/Core_1/Instruction Fetch (IF) Stage ==
  In1 : Inport
  In2 : Inport  Port=2
  Bus Creator : BusCreator  Inputs=2  OutDataTypeStr=Bus: IFID_Bus  NonVirtualBus=on
  Clock : Clock
  Compare To Constant : simulink/Logic and Bit Operations/Compare To Constant  relop=>  const=4.0  OutDataTypeStr=boolean
  Constant : Constant  Value=4
  Constant1 : Constant  Value=0
  Constant2 : Constant  Value=256  OutDataTypeStr=uint32
  Gain : Gain  Gain=0.25  OutDataTypeStr=uint32
  Logical Operator : Logic  AllPortsSameDT=off  OutDataTypeStr=boolean
  Logical Operator1 : Logic  AllPortsSameDT=off  OutDataTypeStr=boolean
  MATLAB Function : MATLAB Function  TreatAsAtomicUnit=on
  Scope1 : Scope
      settings: ActiveDisplayYMinimum=17.53381287399019  ActiveDisplayYMaximum=50.599648083752676  DataLoggingVariableName=ScopeData6
  Sum : Sum  Inputs=|++  OutDataTypeStr=uint32  AccumDataTypeStr=uint32
  Switch : Switch  Criteria=u2 > Threshold  OutDataTypeStr=uint32  SaturateOnIntegerOverflow=off  InputSameDT=off
  Switch1 : Switch  Criteria=u2 > Threshold  OutDataTypeStr=uint32  SaturateOnIntegerOverflow=off  InputSameDT=off
  Switch2 : Switch  Criteria=u2 > Threshold  OutDataTypeStr=uint32  SaturateOnIntegerOverflow=off  InputSameDT=off
  Switch3 : Switch  Criteria=u2 > Threshold  SaturateOnIntegerOverflow=off  InputSameDT=off
  Unit Delay : UnitDelay  HasFrameUpgradeWarning=on
  Out1 : Outport
  Out2 : Outport  Port=2
  tag scope: Flushing1=global
  wires:
  Unit Delay/1 -> Scope1/1, Bus Creator/2, Sum/1, Gain/1  "PC"
  Constant/1 -> Sum/2
  In1/1 -> Switch/3  "Instruction"
  [jump_target_address1] -> Switch2/1
  Logical Operator1/1 -> Switch/2, Switch1/2, [Flushing1]
  Sum/1 -> Switch1/3  "P+4"
  Bus Creator/1 -> Out1/1
  Switch1/1 -> Switch2/3
  Switch2/1 -> Switch3/3
  [Jump1] -> Logical Operator/1
  [Branch_Target_Address1] -> Switch1/1
  Clock/1 -> Compare To Constant/1
  Compare To Constant/1 -> Logical Operator1/2, Logical Operator/2  "Feedback_Enable"
  Logical Operator/1 -> Switch2/2
  [Flush1] -> Logical Operator1/1
  MATLAB Function/1(scalar_out) -> Bus Creator/1  "Instruction"
  Switch/1 -> MATLAB Function/1(vector_in)
  Constant1/1 -> Switch/1
  Gain/1 -> Out2/1
  Switch3/1 -> Unit Delay/1
  Constant2/1 -> Switch3/1
  In2/1 -> Switch3/2

== system processor_with_peripherals/Processor/Core_1/Memory Access ==
  In1 : Inport
  Bus Creator : BusCreator  Inputs=4  OutDataTypeStr=Bus: MEMWB_Bus
  Bus Selector : BusSelector  OutputSignals=read_data_2,ALU_Result,MemWrite,RegWrite,MemRead,rd,AtomicOp
  Switch : Switch  Criteria=u2 > Threshold  SaturateOnIntegerOverflow=off  InputSameDT=off
  Out1 : Outport
  Out2 : Outport  Port=2
  Out3 : Outport  Port=3
  Out4 : Outport  Port=4
  Out5 : Outport  Port=5
  wires:
  In1/1 -> Bus Selector/1
  Bus Selector/2 -> Switch/1, Out2/1, Bus Creator/1  "<ALU_Result>"
  Bus Selector/6 -> Bus Creator/4  "<rd>"
  Bus Selector/3 -> Out5/1  "<MemWrite>"
  Bus Selector/5 -> Bus Creator/3, Out4/1  "<MemRead>"
  Bus Selector/4 -> Bus Creator/2  "<RegWrite>"
  Bus Selector/1 -> Switch/3  "<read_data_2>"
  Bus Creator/1 -> Out1/1
  Switch/1 -> Out3/1
  Bus Selector/7 -> Switch/2  "<AtomicOp>"

== system processor_with_peripherals/Processor/Core_1/Write Back ==
  In1 : Inport
  In2 : Inport  Port=2
  Bus Creator : BusCreator  Inputs=3
  Bus Selector : BusSelector  OutputSignals=ALU_Result,rd,MemRead,RegWrite
  Switch : Switch  Criteria=u2 > Threshold  SaturateOnIntegerOverflow=off  InputSameDT=off
  Out1 : Outport
  wires:
  Bus Creator/1 -> Out1/1
  In1/1 -> Bus Selector/1
  Bus Selector/1 -> Switch/3  "<ALU_Result>"
  Bus Selector/2 -> Bus Creator/2  "<rd>"
  Bus Selector/4 -> Bus Creator/3  "<RegWrite>"
  Bus Selector/3 -> Switch/2  "<MemRead>"
  Switch/1 -> Bus Creator/1  "Switchout"
  In2/1 -> Switch/1

== system processor_with_peripherals/Processor/Core_2/Execute (EX) Stage ==
  In1 : Inport
  Bus Creator : BusCreator  Inputs=7  OutDataTypeStr=Bus: EXMEM_Bus  NonVirtualBus=on
  Bus Selector : BusSelector  OutputSignals=read_data_1,PCSrc,immediate_out,ALUSrc,read_data_2,ALUOp,Instruction,rd,Branch,MemWrite,MemRead,RegWrite,PC,Jump,AtomicOp
  Logical Operator : Logic  AllPortsSameDT=off  OutDataTypeStr=boolean
  Logical Operator1 : Logic  Operator=OR  AllPortsSameDT=off  OutDataTypeStr=boolean
  MATLAB Function : MATLAB Function  TreatAsAtomicUnit=on
  Scope : Scope
      settings: ActiveDisplayYMinimum=-15.043178347449025  ActiveDisplayYMaximum=57.4325180487373
  Scope1 : Scope
      settings: ActiveDisplayYMinimum=91.787947621079041  ActiveDisplayYMaximum=102.5794088339111
  Scope2 : Scope
      settings: ActiveDisplayYMinimum=-11.618054609297872  ActiveDisplayYMaximum=8.6667189404735723  DataLoggingVariableName=ScopeData2
  Sum : Sum  Inputs=|++
  Switch : Switch  Criteria=u2 > Threshold  OutDataTypeStr=int32  SaturateOnIntegerOverflow=off  InputSameDT=off
  Switch1 : Switch  Criteria=u2 > Threshold  OutDataTypeStr=int32  SaturateOnIntegerOverflow=off  InputSameDT=off
  Out1 : Outport
  tag scope: Branch_Target_Address2=global, Flush2=global, Jump2=global, jump_target_address2=global
  wires:
  Bus Creator/1 -> Out1/1
  In1/1 -> Bus Selector/1
  Bus Selector/3 -> Sum/2, Switch/1  "<immediate_out>"
  Bus Selector/8 -> Bus Creator/3  "<rd>"
  Bus Selector/5 -> Bus Creator/2, Switch/3  "<read_data_2>"
  Bus Selector/1 -> Switch1/3  "<read_data_1>"
  Bus Selector/6 -> MATLAB Function/3(ALUOp)  "<ALUOp>"
  Bus Selector/14 -> [Jump2], Logical Operator1/2, Scope2/1  "<Jump>"
  Bus Selector/9 -> Logical Operator/2  "<Branch>"
  Bus Selector/10 -> Bus Creator/4  "<MemWrite>"
  Bus Selector/11 -> Bus Creator/5  "<MemRead>"
  Bus Selector/4 -> Switch/2  "<ALUSrc>"
  Bus Selector/12 -> Bus Creator/6  "<RegWrite>"
  Bus Selector/7 -> MATLAB Function/4(Instruction)  "<Instruction>"
  Switch/1 -> MATLAB Function/2(Operand2)
  MATLAB Function/1(ALU_Result) -> Scope/1, Bus Creator/1, [jump_target_address2]
  MATLAB Function/2(Zero_Flag) -> Logical Operator/1
  Logical Operator/1 -> Logical Operator1/1  "Take_Branch"
  Bus Selector/13 -> Sum/1, Switch1/1  "<PC>"
  Sum/1 -> [Branch_Target_Address2]
  Bus Selector/2 -> Switch1/2  "<PCSrc>"
  Switch1/1 -> Scope1/1, MATLAB Function/1(Operand1)
  Logical Operator1/1 -> [Flush2]
  Bus Selector/15 -> MATLAB Function/5(AtomicOp), Bus Creator/7  "<AtomicOp>"

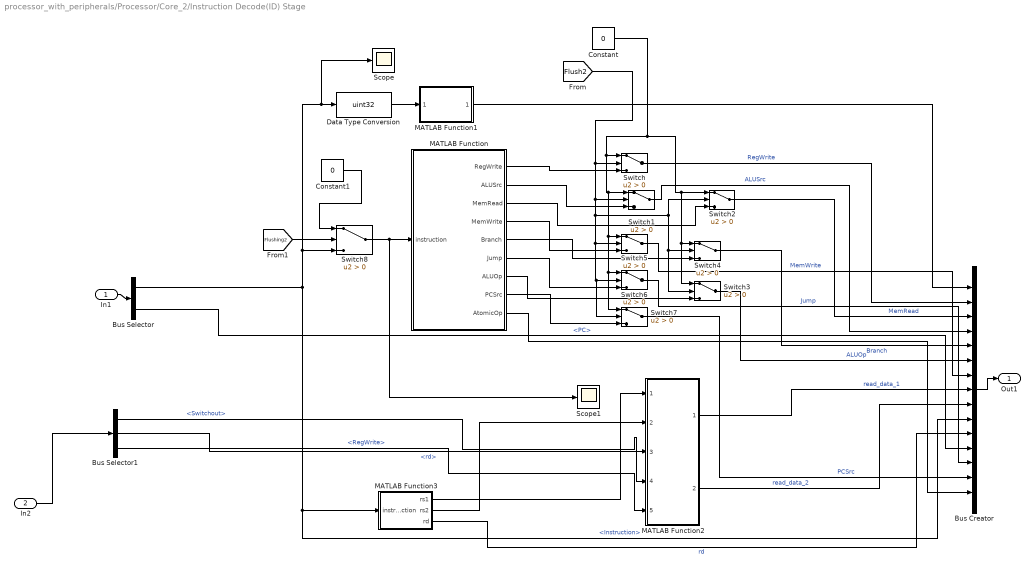
== system processor_with_peripherals/Processor/Core_2/Instruction Decode(ID) Stage ==
  In1 : Inport
  In2 : Inport  Port=2
  Bus Creator : BusCreator  Inputs=15  OutDataTypeStr=Bus: IDEX_Bus  NonVirtualBus=on
  Bus Selector : BusSelector  OutputSignals=Instruction,PC
  Bus Selector1 : BusSelector  OutputSignals=Switchout,rd,RegWrite
  Constant : Constant  Value=0  OutDataTypeStr=uint8
  Constant1 : Constant  Value=0
  Data Type Conversion : DataTypeConversion  OutDataTypeStr=uint32  SaturateOnIntegerOverflow=off  RndMeth=Floor
  MATLAB Function : MATLAB Function  TreatAsAtomicUnit=on
  MATLAB Function1 : MATLAB Function  TreatAsAtomicUnit=on
  MATLAB Function2 : MATLAB Function  TreatAsAtomicUnit=on
  MATLAB Function3 : MATLAB Function  TreatAsAtomicUnit=on
  Scope : Scope
      settings: ActiveDisplayYMinimum=-8.6059552101299882E+7  ActiveDisplayYMaximum=2.8669047582629967E+8  DataLoggingVariableName=ScopeData4
  Scope1 : Scope
      settings: ActiveDisplayYMinimum=-0.20992987297977578  ActiveDisplayYMaximum=4.3440753791982463  DataLoggingVariableName=ScopeData5
  Switch{,1..2,5..6} (5 alike) : Switch  Criteria=u2 > Threshold  OutDataTypeStr=boolean  SaturateOnIntegerOverflow=off  InputSameDT=off
  Switch3 : Switch  Criteria=u2 > Threshold  OutDataTypeStr=uint32  SaturateOnIntegerOverflow=off  InputSameDT=off
  Switch4 : Switch  Criteria=u2 > Threshold  OutDataTypeStr=uint32  SaturateOnIntegerOverflow=off  InputSameDT=off
  Switch7 : Switch  Criteria=u2 > Threshold  OutDataTypeStr=uint32  SaturateOnIntegerOverflow=off  InputSameDT=off
  Switch8 : Switch  Criteria=u2 > Threshold  SaturateOnIntegerOverflow=off  InputSameDT=off
  Out1 : Outport
  wires:
  Bus Creator/1 -> Out1/1
  In1/1 -> Bus Selector/1
  Bus Selector/1 -> Data Type Conversion/1, Scope/1, Switch8/3, MATLAB Function3/1(instruction), Bus Creator/10  "<Instruction>"
  MATLAB Function2/1(ReadData1) -> Bus Creator/8  "read_data_1"
  MATLAB Function2/2(ReadData2) -> Bus Creator/9  "read_data_2"
  MATLAB Function1/1(immediate_out) -> Bus Creator/1
  MATLAB Function3/3(rd) -> Bus Creator/11  "rd"
  MATLAB Function/7(ALUOp) -> Switch3/3
  MATLAB Function/6(Jump) -> Switch6/3
  MATLAB Function/5(Branch) -> Switch4/3
  MATLAB Function/4(MemWrite) -> Switch5/3
  MATLAB Function/3(MemRead) -> Switch2/3
  MATLAB Function/2(ALUSrc) -> Switch1/3
  Bus Selector1/2 -> MATLAB Function2/3(WriteAddr)  "<rd>"
  Bus Selector1/3 -> MATLAB Function2/5(WriteEnable)  "<RegWrite>"
  Bus Selector1/1 -> MATLAB Function2/4(WriteData)  "<Switchout>"
  MATLAB Function3/2(rs2) -> MATLAB Function2/2(ReadAddr2)
  Bus Selector/2 -> Bus Creator/12  "<PC>"
  MATLAB Function/8(PCSrc) -> Switch7/3
  MATLAB Function/1(RegWrite) -> Switch/3
  [Flush2] -> Switch1/2, Switch3/2, Switch4/2, Switch2/2, Switch7/2, Switch6/2, Switch5/2, Switch/2
  Constant/1 -> Switch3/1, Switch4/1, Switch2/1, Switch7/1, Switch6/1, Switch5/1, Switch1/1, Switch/1
  Switch/1 -> Bus Creator/2  "RegWrite"
  Switch2/1 -> Bus Creator/3  "MemRead"
  Switch1/1 -> Bus Creator/4  "ALUSrc"
  Switch4/1 -> Bus Creator/5  "Branch"
  Switch3/1 -> Bus Creator/6  "ALUOp"
  Switch5/1 -> Bus Creator/7  "MemWrite"
  Switch6/1 -> Bus Creator/13  "Jump"
  Switch7/1 -> Bus Creator/14  "PCSrc"
  MATLAB Function3/1(rs1) -> MATLAB Function2/1(ReadAddr1)
  In2/1 -> Bus Selector1/1
  Switch8/1 -> Scope1/1, MATLAB Function/1(instruction)
  Constant1/1 -> Switch8/1
  [Flushing2] -> Switch8/2
  Data Type Conversion/1 -> MATLAB Function1/1(instruction)
  MATLAB Function/9(AtomicOp) -> Bus Creator/15

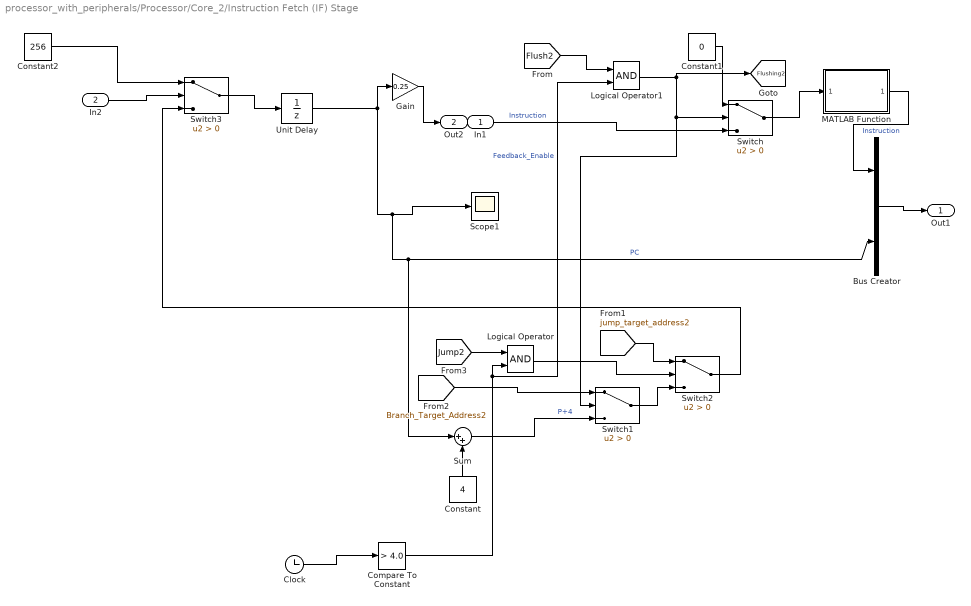
== system processor_with_peripherals/Processor/Core_2/Instruction Fetch (IF) Stage ==
  In1 : Inport
  In2 : Inport  Port=2
  Bus Creator : BusCreator  Inputs=2  OutDataTypeStr=Bus: IFID_Bus  NonVirtualBus=on
  Clock : Clock
  Compare To Constant : simulink/Logic and Bit Operations/Compare To Constant  relop=>  const=4.0  OutDataTypeStr=boolean
  Constant : Constant  Value=4
  Constant1 : Constant  Value=0
  Constant2 : Constant  Value=256  OutDataTypeStr=uint32
  Gain : Gain  Gain=0.25  OutDataTypeStr=uint32
  Logical Operator : Logic  AllPortsSameDT=off  OutDataTypeStr=boolean
  Logical Operator1 : Logic  AllPortsSameDT=off  OutDataTypeStr=boolean
  MATLAB Function : MATLAB Function  TreatAsAtomicUnit=on
  Scope1 : Scope
      settings: ActiveDisplayYMinimum=14.083038013644533  ActiveDisplayYMaximum=56.284353840527714  DataLoggingVariableName=ScopeData6
  Sum : Sum  Inputs=|++  OutDataTypeStr=uint32  AccumDataTypeStr=uint32
  Switch : Switch  Criteria=u2 > Threshold  OutDataTypeStr=uint32  SaturateOnIntegerOverflow=off  InputSameDT=off
  Switch1 : Switch  Criteria=u2 > Threshold  OutDataTypeStr=uint32  SaturateOnIntegerOverflow=off  InputSameDT=off
  Switch2 : Switch  Criteria=u2 > Threshold  OutDataTypeStr=uint32  SaturateOnIntegerOverflow=off  InputSameDT=off
  Switch3 : Switch  Criteria=u2 > Threshold  SaturateOnIntegerOverflow=off  InputSameDT=off
  Unit Delay : UnitDelay  HasFrameUpgradeWarning=on
  Out1 : Outport
  Out2 : Outport  Port=2
  tag scope: Flushing2=global
  wires:
  Unit Delay/1 -> Scope1/1, Bus Creator/2, Sum/1, Gain/1  "PC"
  Constant/1 -> Sum/2
  In1/1 -> Switch/3  "Instruction"
  [jump_target_address2] -> Switch2/1
  Logical Operator1/1 -> Switch/2, Switch1/2, [Flushing2]
  Sum/1 -> Switch1/3  "P+4"
  Bus Creator/1 -> Out1/1
  Switch1/1 -> Switch2/3
  Switch2/1 -> Switch3/3
  [Jump2] -> Logical Operator/1
  [Branch_Target_Address2] -> Switch1/1
  Clock/1 -> Compare To Constant/1
  Compare To Constant/1 -> Logical Operator1/2, Logical Operator/2  "Feedback_Enable"
  Logical Operator/1 -> Switch2/2
  [Flush2] -> Logical Operator1/1
  MATLAB Function/1(scalar_out) -> Bus Creator/1  "Instruction"
  Switch/1 -> MATLAB Function/1(vector_in)
  Constant1/1 -> Switch/1
  Gain/1 -> Out2/1
  Switch3/1 -> Unit Delay/1
  In2/1 -> Switch3/2
  Constant2/1 -> Switch3/1

== system processor_with_peripherals/Processor/Core_2/Memory Access ==
  In1 : Inport
  Bus Creator : BusCreator  Inputs=4  OutDataTypeStr=Bus: MEMWB_Bus
  Bus Selector : BusSelector  OutputSignals=read_data_2,ALU_Result,MemWrite,RegWrite,MemRead,rd,AtomicOp
  Switch : Switch  Criteria=u2 > Threshold  SaturateOnIntegerOverflow=off  InputSameDT=off
  Out1 : Outport
  Out2 : Outport  Port=2
  Out3 : Outport  Port=3
  Out4 : Outport  Port=4
  Out5 : Outport  Port=5
  wires:
  In1/1 -> Bus Selector/1
  Bus Selector/2 -> Switch/1, Out2/1, Bus Creator/1  "<ALU_Result>"
  Bus Selector/6 -> Bus Creator/4  "<rd>"
  Bus Selector/3 -> Out5/1  "<MemWrite>"
  Bus Selector/5 -> Bus Creator/3, Out4/1  "<MemRead>"
  Bus Selector/4 -> Bus Creator/2  "<RegWrite>"
  Bus Selector/1 -> Switch/3  "<read_data_2>"
  Bus Creator/1 -> Out1/1
  Switch/1 -> Out3/1
  Bus Selector/7 -> Switch/2  "<AtomicOp>"

== system processor_with_peripherals/Processor/Core_2/Write Back ==
  In1 : Inport
  In2 : Inport  Port=2
  Bus Creator : BusCreator  Inputs=3
  Bus Selector : BusSelector  OutputSignals=ALU_Result,rd,MemRead,RegWrite
  Switch : Switch  Criteria=u2 > Threshold  SaturateOnIntegerOverflow=off  InputSameDT=off
  Out1 : Outport
  wires:
  Bus Creator/1 -> Out1/1
  In1/1 -> Bus Selector/1
  Bus Selector/1 -> Switch/3  "<ALU_Result>"
  Bus Selector/2 -> Bus Creator/2  "<rd>"
  Bus Selector/4 -> Bus Creator/3  "<RegWrite>"
  Bus Selector/3 -> Switch/2  "<MemRead>"
  Switch/1 -> Bus Creator/1  "Switchout"
  In2/1 -> Switch/1

== system processor_with_peripherals/Processor/Core_3/Execute (EX) Stage ==
  In1 : Inport
  Bus Creator : BusCreator  Inputs=7  OutDataTypeStr=Bus: EXMEM_Bus  NonVirtualBus=on
  Bus Selector : BusSelector  OutputSignals=read_data_1,PCSrc,immediate_out,ALUSrc,read_data_2,ALUOp,Instruction,rd,Branch,MemWrite,MemRead,RegWrite,PC,Jump,AtomicOp
  Logical Operator : Logic  AllPortsSameDT=off  OutDataTypeStr=boolean
  Logical Operator1 : Logic  Operator=OR  AllPortsSameDT=off  OutDataTypeStr=boolean
  MATLAB Function : MATLAB Function  TreatAsAtomicUnit=on
  Scope : Scope
      settings: ActiveDisplayYMinimum=-16.016569239691567  ActiveDisplayYMaximum=60.082911976304075
  Scope1 : Scope
      settings: ActiveDisplayYMinimum=91.787947621079041  ActiveDisplayYMaximum=102.5794088339111
  Scope2 : Scope
      settings: ActiveDisplayYMinimum=-11.618054609297872  ActiveDisplayYMaximum=8.6667189404735723  DataLoggingVariableName=ScopeData2
  Sum : Sum  Inputs=|++
  Switch : Switch  Criteria=u2 > Threshold  OutDataTypeStr=int32  SaturateOnIntegerOverflow=off  InputSameDT=off
  Switch1 : Switch  Criteria=u2 > Threshold  OutDataTypeStr=int32  SaturateOnIntegerOverflow=off  InputSameDT=off
  Out1 : Outport
  tag scope: Branch_Target_Address3=global, Flush3=global, Jump3=global, jump_target_address3=global
  wires:
  Bus Creator/1 -> Out1/1
  In1/1 -> Bus Selector/1
  Bus Selector/3 -> Sum/2, Switch/1  "<immediate_out>"
  Bus Selector/8 -> Bus Creator/3  "<rd>"
  Bus Selector/5 -> Bus Creator/2, Switch/3  "<read_data_2>"
  Bus Selector/1 -> Switch1/3  "<read_data_1>"
  Bus Selector/6 -> MATLAB Function/3(ALUOp)  "<ALUOp>"
  Bus Selector/14 -> [Jump3], Logical Operator1/2, Scope2/1  "<Jump>"
  Bus Selector/9 -> Logical Operator/2  "<Branch>"
  Bus Selector/10 -> Bus Creator/4  "<MemWrite>"
  Bus Selector/11 -> Bus Creator/5  "<MemRead>"
  Bus Selector/4 -> Switch/2  "<ALUSrc>"
  Bus Selector/12 -> Bus Creator/6  "<RegWrite>"
  Bus Selector/7 -> MATLAB Function/4(Instruction)  "<Instruction>"
  Switch/1 -> MATLAB Function/2(Operand2)
  MATLAB Function/1(ALU_Result) -> Scope/1, Bus Creator/1, [jump_target_address3]
  MATLAB Function/2(Zero_Flag) -> Logical Operator/1
  Logical Operator/1 -> Logical Operator1/1  "Take_Branch"
  Bus Selector/13 -> Sum/1, Switch1/1  "<PC>"
  Sum/1 -> [Branch_Target_Address3]
  Bus Selector/2 -> Switch1/2  "<PCSrc>"
  Switch1/1 -> Scope1/1, MATLAB Function/1(Operand1)
  Logical Operator1/1 -> [Flush3]
  Bus Selector/15 -> MATLAB Function/5(AtomicOp), Bus Creator/7  "<AtomicOp>"
